simulink model "Tester_Controller_B"  (R2024b)
settings: Solver=VariableStepAuto  StartTime=0.0  StopTime=inf  RelTol=1e-3
values from neighbouring files (symbols this model uses):
  clegg_mhe = 0.76106    [Lookup_Tables_and_Initializer.m]
  Const_vars2 = Const_vars    [Lookup_Tables_and_Initializer.m]
  cost_1 = 1    [Lookup_Tables_and_Initializer.m]
  cost_2 = 1    [Lookup_Tables_and_Initializer.m]
  D1_mhe = 0.20358    [Lookup_Tables_and_Initializer.m]
  D2_mhe = 0.0098802    [Lookup_Tables_and_Initializer.m]
  E_table = E(V_range2,h_funct(Max_Terminal_V_factor),Sharpness_Const)    [Lookup_Tables.m]    (also in Lookup_Tables_and_Initializer.m)
  I1_mhe = 0.7775    [Lookup_Tables_and_Initializer.m]
  I2_mhe = 0.16299    [Lookup_Tables_and_Initializer.m]
  P1_mhe = 4.742    [Lookup_Tables_and_Initializer.m]
  P2_mhe = 0.25805    [Lookup_Tables_and_Initializer.m]
  Q_table = interp1(PWM,NTF,1000+u_range*13)    [DuoCopter_EOM2.m]    (also in Lookup_Tables.m; Lookup_Tables_and_Initializer.m)
  T_table = zeros(size(V_range))    [DuoCopter_EOM2.m]    (also in Lookup_Tables.m; Lookup_Tables_and_Initializer.m)
  time_horizon = 12    [Lookup_Tables_and_Initializer.m]
  u_range = 0:1:100    [DuoCopter_EOM2.m]    (also in Lookup_Tables.m; Lookup_Tables_and_Initializer.m)
  V_range = linspace(0,1.25,10)    [DuoCopter_EOM2.m]    (also in Lookup_Tables.m; Lookup_Tables_and_Initializer.m)
  V_range2 = 0:0.01:1.44    [Lookup_Tables.m]    (also in Lookup_Tables_and_Initializer.m)
  var_v = 1/0.34    (= 2.94117647059)    [Lookup_Tables_and_Initializer.m]
  var_x = 1/0.015    (= 66.6666666667)    [Lookup_Tables_and_Initializer.m]
  w_k = 0.005    [Lookup_Tables_and_Initializer.m]
  x_bottom = Const(11)    [DT_EOM_fcn2.m]    (also in Lookup_Tables_and_Initializer.m = 0)
  x_top = Const(12)    [DT_EOM_fcn2.m]    (also in Lookup_Tables_and_Initializer.m = 1.44)
undefined symbols (not defined in the file or in its folder): DiscIntNeverNeededParam
libraries: slpidlib x3, simulink x2, instrumentlib x2, dspstat3 x1, dspindex x1, realtime_pacer_lib x1, SignalEditorBlockLib x1
settings Model: Creator=errikos  LastModifiedBy=sh2323
settings SolverCC: AlgebraicLoopSolver=TrustRegion
settings DataIOCC: ReturnWorkspaceOutputs=off
settings DebuggingCC: UnconnectedInputMsg=warning  UnconnectedOutputMsg=warning  UnconnectedLineMsg=warning  ArithmeticOperatorsInVariantConditions=warning
settings ModelReferenceCC: EnableRefExpFcnMdlSchedulingChecks=on
settings SFSimCC: CustomCodeUndefinedFunction=UseInterfaceOnly
settings RTWCC: GPUComputeCapability=3.5  DLArmComputeVersion=19.05

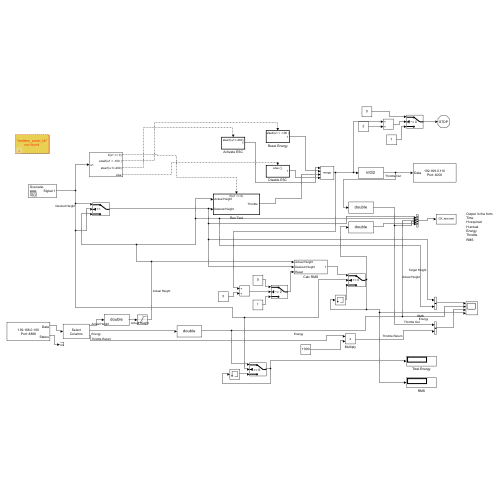
[thumbnail: Simulink's stored preview of the top-level diagram]
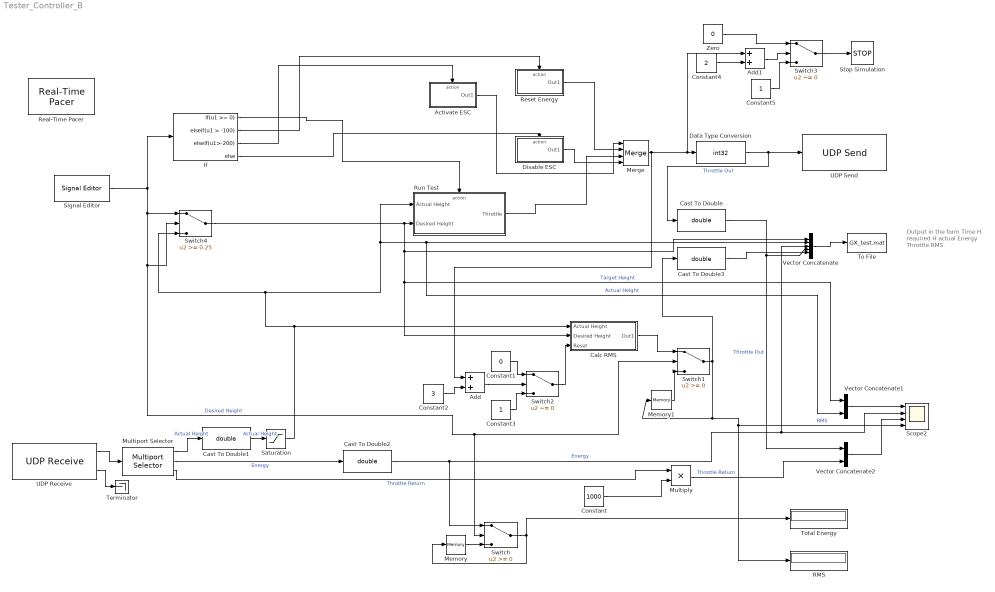
== system Tester_Controller_B ==
  note: Output in the form
      | Time
      | H required
      | H actual
      | Energy
      | Throttle
      | RMS
  Activate ESC : Subsystem  TreatAsAtomicUnit=on
  Add : Sum
  Add1 : Sum
  Calc RMS : Subsystem
  Cast To Double{,1..3} (4 alike) : DataTypeConversion  OutDataTypeStr=double  SaturateOnIntegerOverflow=off  RndMeth=Floor
  Constant : Constant  Value=1000
  Constant1 : Constant  Value=0
  Constant2 : Constant  Value=3
  Constant3 : Constant
  Constant4 : Constant  Value=2
  Constant5 : Constant
  Data Type Conversion : DataTypeConversion  OutDataTypeStr=int32  SaturateOnIntegerOverflow=off  RndMeth=Floor
  Disable ESC : Subsystem  TreatAsAtomicUnit=on
  If : If  IfExpression=u1 >= 0  ElseIfExpressions=u1 > -100 , u1>-200
  Memory : Memory
  Memory1 : Memory
  Merge : Merge  Inputs=4
  Multiply : Product
  Multiport Selector : dspindex/Multiport Selector  rowsOrCols=Columns  idxCellArray={ 1, 2,3}  idxErrMode=Clip and Warn
  RMS : Display
  Real-Time Pacer : realtime_pacer_lib/Real-Time Pacer  simTimePerRealTime=1
  Reset Energy : Subsystem  TreatAsAtomicUnit=on
  Run Test : Subsystem  TreatAsAtomicUnit=on
  Saturation : Saturate  UpperLimit=1.7  LowerLimit=0
  Scope2 : Scope  NumInputPorts=4
  Signal Editor : SignalEditorBlockLib/Signal Editor  FileName=/Users/errikoslevis/Downloads/Simulink Testing/samplemission.mat  ActiveScenario=Scenario  ActiveSignal=Signal 1  IsBus=off  OutputBusObjectStr=Bus: BusObject  SampleTime=0.05  ZeroCross=off  OutputAfterFinalValue=Setting to zero  Unit=inherit  PreserveSignalName=on  ApplySigPropsToAllScenarios=on  ApplySigPropsToAllSignals=off
  Stop Simulation : Stop
  Switch : Switch  SaturateOnIntegerOverflow=off  InputSameDT=off
  Switch1 : Switch  SaturateOnIntegerOverflow=off  InputSameDT=off
  Switch2 : Switch  Criteria=u2 ~= 0  SaturateOnIntegerOverflow=off  InputSameDT=off
  Switch3 : Switch  Criteria=u2 ~= 0  ZeroCross=off  SaturateOnIntegerOverflow=off  InputSameDT=off
  Switch4 : Switch  Threshold=0.25  SaturateOnIntegerOverflow=off  InputSameDT=off
  Terminator : Terminator
  To File : ToFile  Filename=GX_test.mat
  Total Energy : Display
  UDP Receive : instrumentlib/UDP Receive  LocalAddress=192.168.0.100  LocalPort=8888  EnablePortSharing=on  Host=192.168.0.110  Port=4000  GetLatestData=on  DataSize="[1  3]"  DataType=single  ASCIIFormatting=%f%f  Terminator=LF  CustomTerminator=10  ByteOrder=little-endian  EnableBlockingMode=off  Timeout=10  SampleTime=0.05  SimulateUsing=Interpreted execution
  UDP Send : instrumentlib/UDP Send  Host=192.168.0.110  Port=4000  LocalAddress=192.168.0.100  LocalPort=-1  EnablePortSharing=on  OutputDatagramPacketSize=4  ByteOrder=little-endian  EnableBlockingMode=on  SimulateUsing=Interpreted execution
  Vector Concatenate : Concatenate  NumInputs=5
  Vector Concatenate1 : Concatenate
  Vector Concatenate2 : Concatenate
  Zero : Constant  Value=0  OutDataTypeStr=Inherit: Inherit via back propagation
  wires:
  UDP Receive/1 -> Multiport Selector/1
  Multiport Selector/1 -> Cast To Double1/1  "Actual Height"
  Multiport Selector/2 -> Cast To Double2/1  "Energy"
  Run Test/1("Throttle ") -> Merge/3
  Data Type Conversion/1 -> Cast To Double/1, UDP Send/1  "Throttle Out"
  Multiport Selector/3 -> Multiply/1  "Throttle Return"
  Multiply/1 -> Vector Concatenate2/2  "Throttle Return"
  Constant/1 -> Multiply/2
  Signal Editor/1 -> Switch4/2, Switch1/2, Switch/2, Switch4/1, If/1  "Desired Height"
  Merge/1 -> Add/1, Add1/1, Data Type Conversion/1
  Vector Concatenate/1 -> To File/1
  If/1 -> Run Test/Action
  If/2 -> Reset Energy/Action
  If/3 -> Activate ESC/Action
  If/4 -> Disable ESC/Action
  Activate ESC/1(Out1) -> Merge/1
  Disable ESC/1(Out1) -> Merge/4
  Switch/1 -> Memory/1, Total Energy/1
  Cast To Double/1 -> Vector Concatenate2/1, Vector Concatenate/4  "Throttle Out"
  Saturation/1 -> Switch4/3, Run Test/1(Actual Height), Vector Concatenate1/2, Vector Concatenate/2, Calc RMS/1(Actual Height)  "Actual Height"
  Cast To Double2/1 -> Switch/1, Scope2/2, Vector Concatenate/3  "Energy"
  Cast To Double3/1 -> Vector Concatenate/5
  Memory/1 -> Switch/3
  Switch1/1 -> RMS/1, Scope2/4, Memory1/1, Cast To Double3/1  "RMS"
  Memory1/1 -> Switch1/3
  Calc RMS/1(Out1) -> Switch1/1
  Switch2/1 -> Calc RMS/3(Reset)
  Constant1/1 -> Switch2/1
  Constant2/1 -> Add/2
  Add/1 -> Switch2/2
  Constant3/1 -> Switch2/3
  Reset Energy/1(Out1) -> Merge/2
  Switch3/1 -> Stop Simulation/1
  Zero/1 -> Switch3/1
  Add1/1 -> Switch3/2
  Constant4/1 -> Add1/2
  Constant5/1 -> Switch3/3
  Vector Concatenate2/1 -> Scope2/3
  Vector Concatenate1/1 -> Scope2/1
  Switch4/1 -> Vector Concatenate/1, Vector Concatenate1/1, Calc RMS/2(Desired Height), Run Test/2(Desired Height)  "Target Height"
  Cast To Double1/1 -> Saturation/1  "Actual Height"
  UDP Receive/2 -> Terminator/1

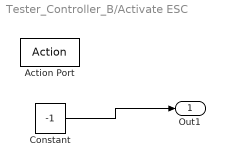
== system Tester_Controller_B/Activate ESC ==
  Action Port : ActionPort  ActionPortLabel=elseif( u1>-200)
  Constant : Constant  Value=-1  SampleTime=0.05
  Out1 : Outport  VectorParamsAs1DForOutWhenUnconnected=off
  wires:
  Constant/1 -> Out1/1

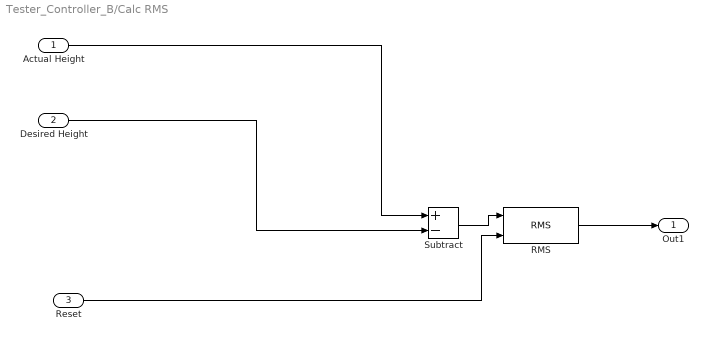
== system Tester_Controller_B/Calc RMS ==
  Actual Height : Inport
  Desired Height : Inport  Port=2
  Reset : Inport  Port=3
  RMS : dspstat3/RMS  run=on  directionMode=Each column  dimension=1  reset_popup=Non-zero sample
  Subtract : Sum  Inputs=+-
  Out1 : Outport  VectorParamsAs1DForOutWhenUnconnected=off
  wires:
  Desired Height/1 -> Subtract/2
  Actual Height/1 -> Subtract/1
  RMS/1 -> Out1/1
  Subtract/1 -> RMS/1
  Reset/1 -> RMS/2

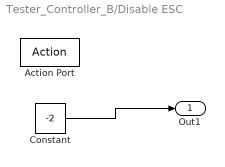
== system Tester_Controller_B/Disable ESC ==
  Action Port : ActionPort  ActionPortLabel=else
  Constant : Constant  Value=-2  SampleTime=0.05
  Out1 : Outport  VectorParamsAs1DForOutWhenUnconnected=off
  wires:
  Constant/1 -> Out1/1

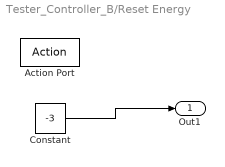
== system Tester_Controller_B/Reset Energy ==
  Action Port : ActionPort  ActionPortLabel=elseif(u1 > -100 )
  Constant : Constant  Value=-3  SampleTime=0.05
  Out1 : Outport  VectorParamsAs1DForOutWhenUnconnected=off
  wires:
  Constant/1 -> Out1/1

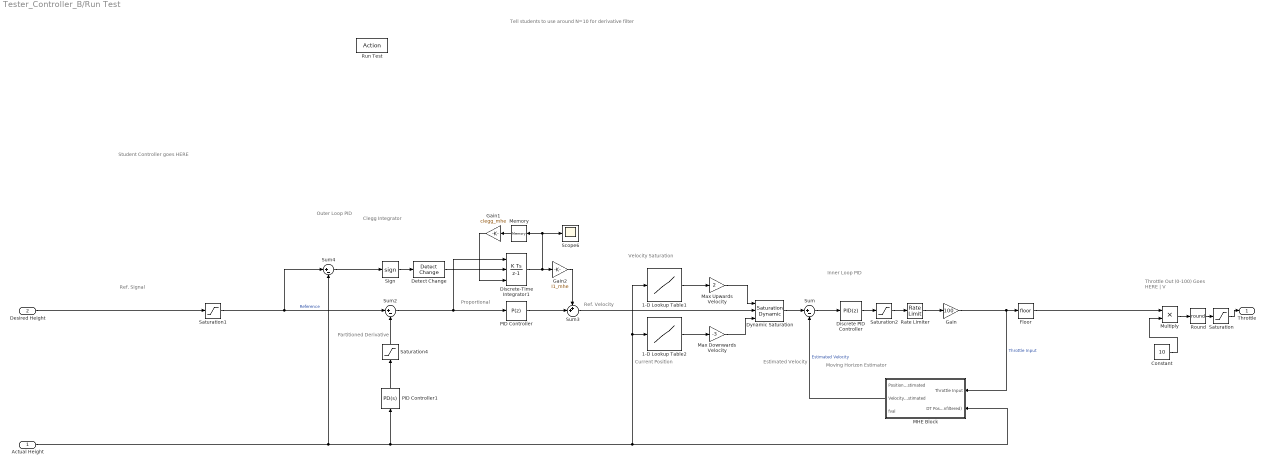
== system Tester_Controller_B/Run Test ==
  note: Tell students to use around N=10 for derivative filter
  note: Throttle Out (0-100)
      | Goes HERE
      |            |
      | 	   V
  note: Student Controller goes HERE
  note: Clegg Integrator
  note: Ref. Signal
  note: Moving Horizon Estimator
  note: Inner Loop PID
  note: Proportional
  note: Velocity Saturation
  note: Outer Loop PID
  note: Estimated Velocity
  note: Partitioned
      | Derivative
  note: Ref. Velocity
  note: Current Position
  Actual Height : Inport
  Desired Height : Inport  Port=2
  Run Test : ActionPort  ActionPortLabel=if(u1 >= 0)
  1-D Lookup Table1 : Lookup_n-D  NumberOfTableDimensions=1  BreakpointsForDimension1=V_range2  Table=flip(E_table)  ExtrapMethod=Clip  InternalRulePriority=Speed  RndMeth=Simplest
  1-D Lookup Table2 : Lookup_n-D  NumberOfTableDimensions=1  BreakpointsForDimension1=V_range2  Table=E_table  ExtrapMethod=Clip  InternalRulePriority=Speed  RndMeth=Simplest
  Constant : Constant  Value=10
  Detect Change : simulink/Logic and Bit Operations/Detect Change  vinit=0  OutDataTypeStr=boolean
  Discrete PID Controller : slpidlib/PID Controller  Controller=PID  Form=Parallel  TimeDomain=Discrete-time  UseExternalTs=off  SampleTime=-1  IntegratorMethod=Forward Euler  FilterMethod=Forward Euler  ControllerParametersSource=internal  P=P2_mhe  I=I2_mhe  UseKiTs=off  D=D2_mhe  UseExternalDerivativeSource=off  N=10  UseFilter=on  TunerSelectOption=Transfer Function Based (PID Tuner App)  InitialConditionSource=internal  InitialConditionForIntegrator=0  InitialConditionForFilter=0  DifferentiatorICPrevScaledInput=0  ExternalReset=none  TrackingMode=off  Kt=1  LimitOutput=on  SatLimitsSource=internal  UpperSaturationLimit=1  LowerSaturationLimit=0  LinearizeAsGain=off  AntiWindupMode=clamping  Kb=1  LimitIntegrator=off  UpperIntegratorSaturationLimit=inf  LowerIntegratorSaturationLimit=-inf  POutMin=[]  POutMax=[]  IOutMin=[]  IOutMax=[]  DOutMin=[]  DOutMax=[]  NOutMin=[]  NOutMax=[]  SumOutMin=[]  SumOutMax=[]  SaturationOutMin=[]  SaturationOutMax=[]  PParamMin=[]  PParamMax=[]  IParamMin=[]  IParamMax=[]  DParamMin=[]  DParamMax=[]  NParamMin=[]  NParamMax=[]  KbParamMin=[]  KbParamMax=[]  KtParamMin=[]  KtParamMax=[]  KbOutMin=[]  KbOutMax=[]  KtOutMin=[]  KtOutMax=[]  IntegratorOutMin=[]  IntegratorOutMax=[]  FilterOutMin=[]  FilterOutMax=[]  SumI1OutMin=[]  SumI1OutMax=[]  SumI2OutMin=[]  SumI2OutMax=[]  SumI3OutMin=[]  SumI3OutMax=[]  SumI4OutMin=[]  SumI4OutMax=[]  SumDOutMin=[]  SumDOutMax=[]  DifferentiatorOutMin=[]  DifferentiatorOutMax=[]  FilterDiffOutCoefMin=[]  FilterDiffOutCoefMax=[]  ReciprocalOutMin=[]  ReciprocalOutMax=[]  SumDenOutMin=[]  SumDenOutMax=[]  SumNumOutMin=[]  SumNumOutMax=[]  DivideOutMin=[]  DivideOutMax=[]  UdiffTsProdOutMin=[]  UdiffTsProdOutMax=[]  NTsProdOutMin=[]  NTsProdOutMax=[]  UintegralTsProdOutMin=[]  UintegralTsProdOutMax=[]  UngainTsProdOutMin=[]  UngainTsProdOutMax=[]  ClampingZeroOutDataTypeStr=Inherit: Inherit via back propagation  ClampingZeroOutMin=[]  ClampingZeroOutMax=[]  FilterDenConstantOutDataTypeStr=Inherit: Inherit via back propagation  FilterDenConstantOutMin=[]  FilterDenConstantOutMax=[]  PCopyOutDataTypeStr=Inherit: Inherit via back propagation  PCopyOutMin=[]  PCopyOutMax=[]  NCopyOutDataTypeStr=Inherit: Inherit via back propagation  NCopyOutMin=[]  NCopyOutMax=[]  IntegratorContinuousStateAttributes=''  IntegratorStateMustResolveToSignalObject=off  IntegratorRTWStateStorageClass=Auto  FilterContinuousStateAttributes=''  FilterStateMustResolveToSignalObject=off  FilterRTWStateStorageClass=Auto  ParallelPVariant=InternalParameters  IdealPVariant=Disabled  IVariant=InternalParameters  DVariant=InternalParameters  IntegratorVariant=Discrete  SatVariant=Enabled  AWVariant=DiscClampingParallel  PCopyVariant=Disabled  TRVariant=Disabled  FdbkBlocksVariant=Forward  IdealPFdbkVariant=Disabled  SatFdbkVariant=Disabled  DerivativeFilterVariant=ForwardEulerFilter  NVariant=InternalParameters  NCopyVariant=Disabled  FilterICVariant=InternalICsFilter  IntegratorICVariant=InternalICs  ExternalResetVariant=Disabled  TRSumVariant=Passthrough  SumFdbkVariant=Disabled  SumVariant=Sum_PID  TsampFilterVariant=InternalTs  TsampNgainVariant=Passthrough  TsampIntegralVariant=Disabled_SignalSpec  ExternalSaturationOutDataTypeStr=Inherit: Same as second input  DerivativeSourceVariant=ErrorSignal  PreIntVariant=InternalPreInt
      settings: LibrarySourceBlock=simulink/Discrete/Discrete PID Controller
  Discrete-Time Integrator1 : DiscreteIntegrator  ExternalReset=level  InitialConditionSource=external  SampleTime=-1  ICPrevOutput=DiscIntNeverNeededParam  ICPrevScaledInput=DiscIntNeverNeededParam
  Dynamic Saturation : simulink/Discontinuities/Saturation Dynamic  OutMin=[]  OutMax=[]  OutDataTypeStr=Inherit: Same as second input  OutDataType=fixdt(1, 16)  OutScaling=2^-10  DoSatur=off
  Floor : Rounding
  Gain : Gain  Gain=100
  Gain1 : Gain  Gain=clegg_mhe
  Gain2 : Gain  Gain=I1_mhe
  MHE Block : Subsystem
  Max Downwards Velocity : Gain  Gain=-3
  Max Upwards Velocity : Gain  Gain=2
  Memory : Memory
  Multiply : Product
  PID Controller : slpidlib/PID Controller  Controller=P  Form=Parallel  TimeDomain=Discrete-time  UseExternalTs=off  SampleTime=-1  IntegratorMethod=Forward Euler  FilterMethod=Forward Euler  ControllerParametersSource=internal  P=P1_mhe  I=4  UseKiTs=off  D=0  UseExternalDerivativeSource=off  N=10  UseFilter=on  TunerSelectOption=Transfer Function Based (PID Tuner App)  InitialConditionSource=internal  InitialConditionForIntegrator=0  InitialConditionForFilter=0  DifferentiatorICPrevScaledInput=0  ExternalReset=none  TrackingMode=off  Kt=1  LimitOutput=off  SatLimitsSource=internal  UpperSaturationLimit=inf  LowerSaturationLimit=-inf  LinearizeAsGain=on  AntiWindupMode=none  Kb=1  LimitIntegrator=off  UpperIntegratorSaturationLimit=inf  LowerIntegratorSaturationLimit=-inf  POutMin=[]  POutMax=[]  IOutMin=[]  IOutMax=[]  DOutMin=[]  DOutMax=[]  NOutMin=[]  NOutMax=[]  SumOutMin=[]  SumOutMax=[]  SaturationOutMin=[]  SaturationOutMax=[]  PParamMin=[]  PParamMax=[]  IParamMin=[]  IParamMax=[]  DParamMin=[]  DParamMax=[]  NParamMin=[]  NParamMax=[]  KbParamMin=[]  KbParamMax=[]  KtParamMin=[]  KtParamMax=[]  KbOutMin=[]  KbOutMax=[]  KtOutMin=[]  KtOutMax=[]  IntegratorOutMin=[]  IntegratorOutMax=[]  FilterOutMin=[]  FilterOutMax=[]  SumI1OutMin=[]  SumI1OutMax=[]  SumI2OutMin=[]  SumI2OutMax=[]  SumI3OutMin=[]  SumI3OutMax=[]  SumI4OutMin=[]  SumI4OutMax=[]  SumDOutMin=[]  SumDOutMax=[]  DifferentiatorOutMin=[]  DifferentiatorOutMax=[]  FilterDiffOutCoefMin=[]  FilterDiffOutCoefMax=[]  ReciprocalOutMin=[]  ReciprocalOutMax=[]  SumDenOutMin=[]  SumDenOutMax=[]  SumNumOutMin=[]  SumNumOutMax=[]  DivideOutMin=[]  DivideOutMax=[]  UdiffTsProdOutMin=[]  UdiffTsProdOutMax=[]  NTsProdOutMin=[]  NTsProdOutMax=[]  UintegralTsProdOutMin=[]  UintegralTsProdOutMax=[]  UngainTsProdOutMin=[]  UngainTsProdOutMax=[]  ClampingZeroOutDataTypeStr=Inherit: Inherit via back propagation  ClampingZeroOutMin=[]  ClampingZeroOutMax=[]  FilterDenConstantOutDataTypeStr=Inherit: Inherit via back propagation  FilterDenConstantOutMin=[]  FilterDenConstantOutMax=[]  PCopyOutDataTypeStr=Inherit: Inherit via back propagation  PCopyOutMin=[]  PCopyOutMax=[]  NCopyOutDataTypeStr=Inherit: Inherit via back propagation  NCopyOutMin=[]  NCopyOutMax=[]  IntegratorContinuousStateAttributes=''  IntegratorStateMustResolveToSignalObject=off  IntegratorRTWStateStorageClass=Auto  FilterContinuousStateAttributes=''  FilterStateMustResolveToSignalObject=off  FilterRTWStateStorageClass=Auto  ParallelPVariant=InternalParameters  IdealPVariant=Disabled  IVariant=Disabled  DVariant=Disabled  IntegratorVariant=Disabled  SatVariant=Disabled  AWVariant=Disabled  PCopyVariant=Disabled  TRVariant=Disabled  FdbkBlocksVariant=Forward  IdealPFdbkVariant=Disabled  SatFdbkVariant=Disabled  DerivativeFilterVariant=Disabled  NVariant=Disabled  NCopyVariant=Disabled_SignalSpec  FilterICVariant=Disabled  IntegratorICVariant=Disabled  ExternalResetVariant=Disabled  TRSumVariant=Passthrough  SumFdbkVariant=Disabled  SumVariant=Passthrough_P  TsampFilterVariant=InternalTs  TsampNgainVariant=Passthrough  TsampIntegralVariant=Disabled_SignalSpec  ExternalSaturationOutDataTypeStr=Inherit: Same as second input  DerivativeSourceVariant=Disabled  PreIntVariant=InternalPreInt
  PID Controller1 : slpidlib/PID Controller  Controller=PD  Form=Parallel  TimeDomain=Continuous-time  UseExternalTs=off  SampleTime=-1  IntegratorMethod=Forward Euler  FilterMethod=Forward Euler  ControllerParametersSource=internal  P=1  I=1  UseKiTs=off  D=D1_mhe/P1_mhe  UseExternalDerivativeSource=off  N=10  UseFilter=on  TunerSelectOption=Transfer Function Based (PID Tuner App)  InitialConditionSource=internal  InitialConditionForIntegrator=0  InitialConditionForFilter=0  DifferentiatorICPrevScaledInput=0  ExternalReset=none  TrackingMode=off  Kt=1  LimitOutput=off  SatLimitsSource=internal  UpperSaturationLimit=inf  LowerSaturationLimit=-inf  LinearizeAsGain=on  AntiWindupMode=none  Kb=1  LimitIntegrator=off  UpperIntegratorSaturationLimit=inf  LowerIntegratorSaturationLimit=-inf  POutMin=[]  POutMax=[]  IOutMin=[]  IOutMax=[]  DOutMin=[]  DOutMax=[]  NOutMin=[]  NOutMax=[]  SumOutMin=[]  SumOutMax=[]  SaturationOutMin=[]  SaturationOutMax=[]  PParamMin=[]  PParamMax=[]  IParamMin=[]  IParamMax=[]  DParamMin=[]  DParamMax=[]  NParamMin=[]  NParamMax=[]  KbParamMin=[]  KbParamMax=[]  KtParamMin=[]  KtParamMax=[]  KbOutMin=[]  KbOutMax=[]  KtOutMin=[]  KtOutMax=[]  IntegratorOutMin=[]  IntegratorOutMax=[]  FilterOutMin=[]  FilterOutMax=[]  SumI1OutMin=[]  SumI1OutMax=[]  SumI2OutMin=[]  SumI2OutMax=[]  SumI3OutMin=[]  SumI3OutMax=[]  SumI4OutMin=[]  SumI4OutMax=[]  SumDOutMin=[]  SumDOutMax=[]  DifferentiatorOutMin=[]  DifferentiatorOutMax=[]  FilterDiffOutCoefMin=[]  FilterDiffOutCoefMax=[]  ReciprocalOutMin=[]  ReciprocalOutMax=[]  SumDenOutMin=[]  SumDenOutMax=[]  SumNumOutMin=[]  SumNumOutMax=[]  DivideOutMin=[]  DivideOutMax=[]  UdiffTsProdOutMin=[]  UdiffTsProdOutMax=[]  NTsProdOutMin=[]  NTsProdOutMax=[]  UintegralTsProdOutMin=[]  UintegralTsProdOutMax=[]  UngainTsProdOutMin=[]  UngainTsProdOutMax=[]  ClampingZeroOutDataTypeStr=Inherit: Inherit via back propagation  ClampingZeroOutMin=[]  ClampingZeroOutMax=[]  FilterDenConstantOutDataTypeStr=Inherit: Inherit via back propagation  FilterDenConstantOutMin=[]  FilterDenConstantOutMax=[]  PCopyOutDataTypeStr=Inherit: Inherit via back propagation  PCopyOutMin=[]  PCopyOutMax=[]  NCopyOutDataTypeStr=Inherit: Inherit via back propagation  NCopyOutMin=[]  NCopyOutMax=[]  IntegratorContinuousStateAttributes=''  IntegratorStateMustResolveToSignalObject=off  IntegratorRTWStateStorageClass=Auto  FilterContinuousStateAttributes=''  FilterStateMustResolveToSignalObject=off  FilterRTWStateStorageClass=Auto  ParallelPVariant=InternalParameters  IdealPVariant=Disabled  IVariant=Disabled  DVariant=InternalParameters  IntegratorVariant=Disabled  SatVariant=Disabled  AWVariant=Disabled  PCopyVariant=Disabled  TRVariant=Disabled  FdbkBlocksVariant=Forward  IdealPFdbkVariant=Disabled  SatFdbkVariant=Disabled  DerivativeFilterVariant=ContFilter  NVariant=InternalParameters  NCopyVariant=Disabled  FilterICVariant=InternalICsFilter  IntegratorICVariant=Disabled  ExternalResetVariant=Disabled  TRSumVariant=Passthrough  SumFdbkVariant=Disabled  SumVariant=Sum_PD  TsampFilterVariant=InternalTs  TsampNgainVariant=Passthrough  TsampIntegralVariant=Disabled_SignalSpec  ExternalSaturationOutDataTypeStr=Inherit: Same as second input  DerivativeSourceVariant=ErrorSignal  PreIntVariant=InternalPreInt
  Rate Limiter : RateLimiter  RisingSlewLimit=4  FallingSlewLimit=-4  SampleTimeMode=inherited
  Round : Rounding  Operator=round
  Saturation : Saturate  UpperLimit=1000  LowerLimit=0
  Saturation1 : Saturate  UpperLimit=x_top  LowerLimit=x_bottom
  Saturation2 : Saturate  UpperLimit=0.9  LowerLimit=0
  Saturation4 : Saturate  UpperLimit=x_top  LowerLimit=x_bottom
  Scope6 : Scope
  Sign : Signum
  Sum : Sum  Inputs=|+-
  Sum2 : Sum  Inputs=|+-
  Sum3 : Sum  Inputs=++|
  Sum4 : Sum  Inputs=|+-
  "Throttle " : Outport  VectorParamsAs1DForOutWhenUnconnected=off
  wires:
  Saturation/1 -> "Throttle "/1
  Constant/1 -> Multiply/2
  Multiply/1 -> Round/1
  Round/1 -> Saturation/1
  PID Controller1/1 -> Saturation4/1
  Saturation1/1 -> Sum2/1, Sum4/1  "Reference"
  Discrete PID Controller/1 -> Saturation2/1
  Saturation2/1 -> Rate Limiter/1
  Rate Limiter/1 -> Gain/1
  Sum4/1 -> Sign/1
  Gain/1 -> Floor/1, MHE Block/1(Throttle Input)  "Throttle Input"
  Dynamic Saturation/1 -> Sum/1
  Gain2/1 -> Sum3/1
  PID Controller/1 -> Sum3/2
  Sum/1 -> Discrete PID Controller/1
  Saturation4/1 -> Sum2/2
  Memory/1 -> Gain1/1
  Max Upwards Velocity/1 -> Dynamic Saturation/1
  Discrete-Time Integrator1/1 -> Memory/1, Scope6/1, Gain2/1
  1-D Lookup Table1/1 -> Max Upwards Velocity/1
  Max Downwards Velocity/1 -> Dynamic Saturation/3
  Floor/1 -> Multiply/1
  Detect Change/1 -> Discrete-Time Integrator1/2
  1-D Lookup Table2/1 -> Max Downwards Velocity/1
  Sum2/1 -> PID Controller/1, Discrete-Time Integrator1/1
  MHE Block/2(Velocity Estimated) -> Sum/2  "Estimated Velocity"
  Gain1/1 -> Discrete-Time Integrator1/3
  Sum3/1 -> Dynamic Saturation/2
  Sign/1 -> Detect Change/1
  Actual Height/1 -> Sum4/2, MHE Block/2(DT Position (Unfiltered)), 1-D Lookup Table1/1, 1-D Lookup Table2/1, PID Controller1/1
  Desired Height/1 -> Saturation1/1

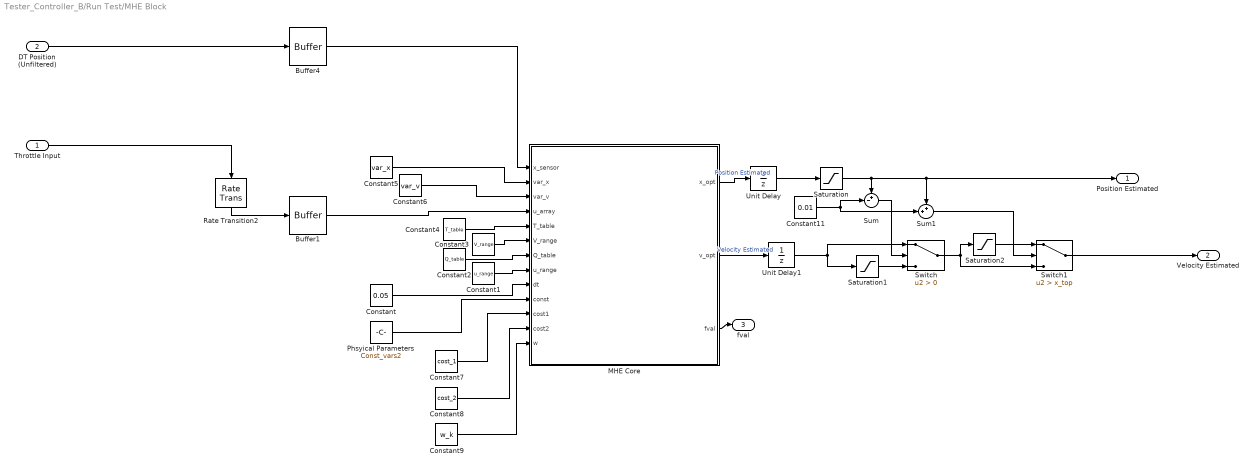
== system Tester_Controller_B/Run Test/MHE Block ==
  Throttle Input : Inport
  DT Position (Unfiltered) : Inport  Port=2
  Buffer1 : Buffer  N=time_horizon  V=time_horizon-1  OutputFrames=off
  Buffer4 : Buffer  N=time_horizon  V=time_horizon-1  OutputFrames=off
  Constant : Constant  Value=0.05
  Constant1 : Constant  Value=u_range
  Constant11 : Constant  Value=0.01
  Constant2 : Constant  Value=Q_table
  Constant3 : Constant  Value=V_range
  Constant4 : Constant  Value=T_table
  Constant5 : Constant  Value=var_x
  Constant6 : Constant  Value=var_v
  Constant7 : Constant  Value=cost_1
  Constant8 : Constant  Value=cost_2
  Constant9 : Constant  Value=w_k
  MHE Core : MATLAB Function  TreatAsAtomicUnit=on
  Phsyical Parameters : Constant  Value=Const_vars2
  Rate Transition2 : RateTransition  OutPortSampleTime=0.05
  Saturation : Saturate  UpperLimit=x_top  LowerLimit=x_bottom
  Saturation1 : Saturate  UpperLimit=inf  LowerLimit=0
  Saturation2 : Saturate  UpperLimit=0  LowerLimit=-inf
  Sum : Sum  Inputs=+-|
  Sum1 : Sum  Inputs=++|
  Switch : Switch  Criteria=u2 > Threshold  SaturateOnIntegerOverflow=off  InputSameDT=off
  Switch1 : Switch  Criteria=u2 > Threshold  Threshold=x_top  SaturateOnIntegerOverflow=off  InputSameDT=off
  Unit Delay : UnitDelay  SampleTime=-1  HasFrameUpgradeWarning=on
  Unit Delay1 : UnitDelay  SampleTime=-1  HasFrameUpgradeWarning=on
  Position Estimated : Outport
  Velocity Estimated : Outport  Port=2
  fval : Outport  Port=3
  wires:
  Constant2/1 -> MHE Core/7(Q_table)
  Rate Transition2/1 -> Buffer1/1
  Constant4/1 -> MHE Core/5(T_table)
  Constant1/1 -> MHE Core/8(u_range)
  Constant6/1 -> MHE Core/3(var_v)
  Constant/1 -> MHE Core/9(dt)
  Constant5/1 -> MHE Core/2(var_x)
  Constant3/1 -> MHE Core/6(V_range)
  Buffer4/1 -> MHE Core/1(x_sensor)
  Buffer1/1 -> MHE Core/4(u_array)
  MHE Core/2(v_opt) -> Unit Delay1/1  "Velocity Estimated"
  DT Position (Unfiltered)/1 -> Buffer4/1
  Throttle Input/1 -> Rate Transition2/1
  MHE Core/3(fval) -> fval/1
  MHE Core/1(x_opt) -> Unit Delay/1  "Position Estimated"
  Unit Delay/1 -> Saturation/1
  Phsyical Parameters/1 -> MHE Core/10(const)
  Constant7/1 -> MHE Core/11(cost1)
  Constant8/1 -> MHE Core/12(cost2)
  Constant9/1 -> MHE Core/13(w)
  Saturation/1 -> Sum/1, Sum1/1, Position Estimated/1
  Saturation1/1 -> Switch/3
  Sum/1 -> Switch/2
  Constant11/1 -> Sum/2, Sum1/2
  Unit Delay1/1 -> Saturation1/1, Switch/1
  Switch/1 -> Switch1/3, Saturation2/1
  Switch1/1 -> Velocity Estimated/1
  Sum1/1 -> Switch1/2
  Saturation2/1 -> Switch1/1

== matlab function Tester_Controller_B/Run Test/MHE Block/MHE Core ==
  data: x_sensor input size=[time_horizon,1]; x_opt output double size=1; var_x input; var_v input; u_array input; T_table input; V_range input; Q_table input; u_range input; dt input; v_opt output double size=1; fval output; const input; cost1 input; cost2 input; w input
function [x_opt, v_opt, fval] = nonlinear_estimator4(x_sensor, var_x, var_v, u_array, T_table, V_range, Q_table, u_range, dt, const, cost1,cost2, w)
    n = length(x_sensor);
    
    x_sensor = x_sensor';
    u_array = u_array';


    % Dynamics function (vectorized)
    h = @(v,x,u) DT_EOM_fcn2(v, x, u, T_table, V_range, Q_table, u_range, dt, const);
    
    % Initial guess (smoothed velocity)

    v_init = diff(x_sensor) / dt;
    v_init = [v_init, v_init(end)]'; % pad last element to length n
    
    z0 = [v_init; x_sensor(:)];
    
    % Objective function (weighted residuals)
    objfun = @(z) ...
        cost1*sum( (x_sensor - z(n+1:end)').^2 / var_x ) + ...  % Measurement residuals
        cost2*sum( (z(2:n) - z(1:n-1) ).^2 / var_v );          % Velocity smoothness
    
    % Nonlinear constraints: Enforce dynamics
    nonlcon = @(z) dynamics_constraints(z, n, u_array, h,w);
    
    % Solver options
    options = optimoptions('fmincon', 'Display', 'iter', 'Algorithm', 'sqp');
    
    % Solve MHE
    [z_opt, fval] = fmincon(objfun, z0, [], [], [], [], [], [], nonlcon, options);
    
    % Extract estimates
    %v_opt = z_opt(1:n);
    %x_opt = z_opt(n+1:end);

    v_opt = z_opt(n);
    x_opt = z_opt(end);
end

% Nonlinear constraints to enforce dynamics


function [c, ceq] = dynamics_constraints(z, n, u_array, h, w)
    % Inputs:
    %   z: decision variables [v; x]
    %   n: number of time steps
    %   u_array: control inputs (vector of size n-1)
    %   h: dynamics function (returns [v_next; x_next])
    %   epsilon: max allowed deviation (scalar or vector)
    
    v = z(1:n);
    x = z(n+1:end);
    c = zeros(4*(n-1), 1);  % 2 inequalities per state (upper/lower bounds)
    
    for i = 1:n-1
        x_next_nominal = h(v(i), x(i), u_array(i));
        
        % Split abs(deviation) ≤ ε into two inequalities:
        %    -ε ≤ (v_next - v_nominal) ≤ ε
        %    -ε ≤ (x_next - x_nominal) ≤ ε
        
        % Velocity constraints (2 inequalities)
        c(4*(i-1)+1) = (v(i+1) - x_next_nominal(1)) - w;
        c(4*(i-1)+2) = -(v(i+1) - x_next_nominal(1)) - w;
        
        % Position constraints (2 inequalities)
        c(4*(i-1)+3) = (x(i+1) - x_next_nominal(2)) - w;
        c(4*(i-1)+4) = -(x(i+1) - x_next_nominal(2)) - w;
    end
    
    ceq = [];  % No equality constraints
end
